simulink model "Modell_Slider_Regelung_Final"  (R2023a)
settings: Solver=FixedStepDiscrete  StartTime=0.0  StopTime=inf  FixedStep=0.1  RelTol=1e-3  EnableMultiTasking=on
model workspace (MAT data in the model file):
  value = 333.2859
undefined symbols (not defined in the file): HIL
libraries: quarc_library x4
settings Model: ExtModeTrigDuration=10000  Creator=Student  LastModifiedBy=Student
settings SolverCC: AlgebraicLoopSolver=TrustRegion  PositivePriorityOrder=on
settings DataIOCC: ReturnWorkspaceOutputs=off
settings DebuggingCC: UnconnectedInputMsg=warning  UnconnectedOutputMsg=warning  UnconnectedLineMsg=warning  ArithmeticOperatorsInVariantConditions=warning
settings ModelReferenceCC: EnableRefExpFcnMdlSchedulingChecks=on
settings SFSimCC: SimUseLocalCustomCode=off  CustomCodeUndefinedFunction=UseInterfaceOnly
settings RTWCC: Description=QUARC Win64 Target Using Toolchain  SystemTargetFile=quarc_win64.tlc  TemplateMakefile=quarc_default_tmf  RTWUseLocalCustomCode=off  Toolchain=QUARC win64 | nmake (64-bit Windows)  BuildConfiguration=Faster Runs
settings CodeAppCC: StateflowObjectComments=on
settings STFCustomTargetCC: SystemTargetFile=quarc_win64.tlc
settings GRTTargetCC: ParMdlRefBuildCompliant=off  CompOptLevelCompliant=off  CombineOutputUpdateFcns=off  MatFileLogging=off  CPPClassGenCompliant=off  GRTInterface=on  ExtMode=on  ExtModeMexFile=quarc_comm
settings ConfigComp: CovMetricSettings=dswe

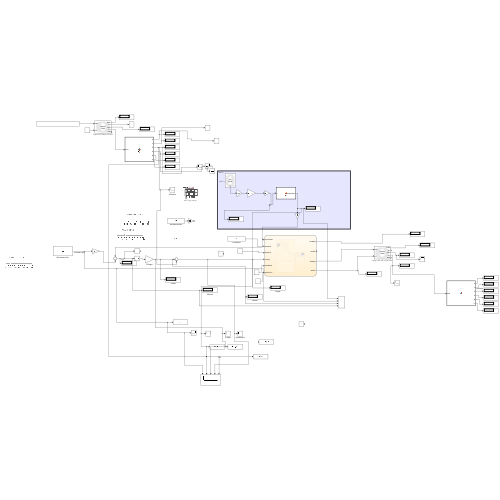
[thumbnail: Simulink's stored preview of the top-level diagram]
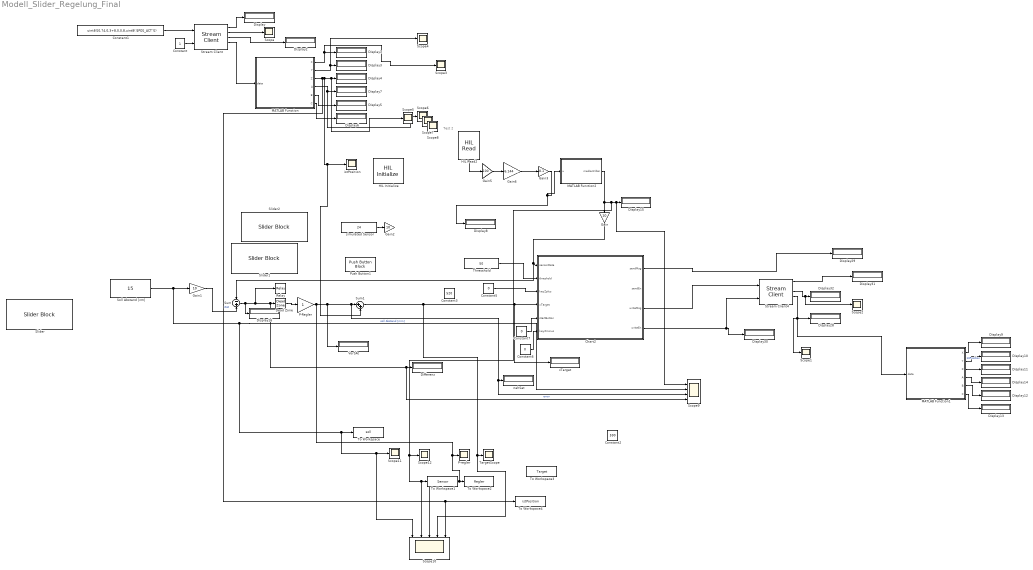
== system Modell_Slider_Regelung_Final ==
  note: Test 2
  Chart2 : Stateflow chart  TreatAsAtomicUnit=on
      settings: PortSchema="{\"entries\":[{\"content\":{\"sides\":[{\"content\":{\"connectorIds\":[\"In1\",\"In6\",\"In2\",\"In3\",\"In4\",\"In5\"]},\"type\":\"ConnectorPlacement.EquallySpacedRectSide\",\"uuid\":\"51d190bc-faf9-4413-9262-a39a5d664301\"},{\"content\":{\"connectorIds\":[\"Out1\",\"Out2\",\"Out3\",\"Out4\"],\"side\":\"RIGHT\"},\"type\":\"ConnectorPlacement.EquallySpacedRectSide\",\"uuid\":\"e4e93cb2-356d-4976-90dd-4fcabb178b84\"},{\"content\":{\"side\":\"TOP\"},\"type\":\"ConnectorPlacement.EquallySpacedRectSide\",\"uuid\":\"2a648fa8-8c40-468b-82f7-fe4bda6b12e2\"}]},\"type\":\"ConnectorPlacement.EquallySpacedConnector\",\"uuid\":\"c42a36e0-454c-4187-a45e-762c1b87647d\"}],\"packageUris\":[\"http://schema.mathworks.com/mf0/Connector/R2020b\"],\"version\":\"1.0\"}"
  Constant : Constant
  Constant1 : Constant  Value=uint8([0,74,0,3+8,0,0,8,uint8('$POS_ACT')])  OutDataTypeStr=uint8
  Constant2 : Constant  Value=590
  Constant3 : Constant  Value=520
  Constant5 : Constant  Value=0  OutDataTypeStr=boolean
  Constant6 : Constant  Value=0  OutDataTypeStr=boolean
  Constant7 : Constant  Value=0
  Dead Zone : DeadZone  LowerValue=-10  UpperValue=10
  Differenz : Display
  Display{,1..16,28..32} (22 alike) : Display
  Gain : Gain  Gain=10
  Gain1 : Gain  Gain=10
  Gain2 : Gain  Gain=10
  Gain3 : Gain  Gain=0.1
  Gain5 : Gain  Gain=100
  Gain6 : Gain  Gain=6.144
  HIL Initialize : quarc_library/Data Acquisition/Generic/Configuration/HIL Initialize  object_name=HIL-1  board_type=q2_usb  board_number=0  board_options=d0=digital;d1=digital;led=auto;update_rate=normal;decimation=1  exclusive=off  active=on  hardware_clocks=[0]  clock_modes=[]  initial_clock_frequencies=[]  set_clock_params_at_start=off  set_clock_params_at_switch_in=off  set_clock_frequencies_at_start=off  set_clock_frequencies_at_switch_in=off  analog_input_channels=[0:1]  analog_input_configurations=[]  analog_input_maximums=10  analog_input_minimums=-10  set_analog_input_params_at_start=on  set_analog_input_params_at_switch_in=off  analog_output_channels=[0:1]  analog_output_maximums=10  analog_output_minimums=-10  initial_analog_outputs=[0]  final_analog_outputs=[0]  watchdog_analog_outputs=0  set_analog_output_params_at_start=on  set_analog_output_params_at_switch_in=off  set_analog_outputs_at_start=on  set_analog_outputs_at_switch_in=off  set_analog_outputs_at_terminate=on  set_analog_outputs_at_switch_out=off  set_analog_outputs_on_watchdog=off  digital_input_channels=[]  digital_output_channels=[]  digital_output_configuration=[]  initial_digital_outputs=[1]  final_digital_outputs=[1]  watchdog_digital_outputs=[1]  set_digital_output_params_at_start=off  set_digital_output_params_at_switch_in=off  set_digital_outputs_at_start=on  set_digital_outputs_at_switch_in=off  set_digital_outputs_at_terminate=on  set_digital_outputs_at_switch_out=off  set_digital_outputs_on_watchdog=off  encoder_channels=[0:1]  quadrature=[4]  encoder_filter_frequency=[]  initial_encoder_counts=[0]  set_encoder_params_at_start=on  set_encoder_params_at_switch_in=off  set_encoder_counts_at_start=on  set_encoder_counts_at_switch_in=off  pwm_channels=[]  pwm_modes=[0]  pwm_frequency=1/0.020  pwm_configuration=[]  pwm_alignment=[]  pwm_polarity=[]  pwm_leading_deadband=[]  pwm_trailing_deadband=[]  initial_pwm_outputs=[0]  final_pwm_outputs=[0]  watchdog_pwm_outputs=[0]  set_pwm_params_at_start=on  set_pwm_params_at_switch_in=off  set_pwm_outputs_at_start=on  set_pwm_outputs_at_switch_in=off  set_pwm_outputs_at_terminate=on  set_pwm_outputs_at_switch_out=off  set_pwm_outputs_on_watchdog=off  other_output_channels=[]  initial_other_outputs=[]  final_other_outputs=[]  watchdog_other_outputs=[]  set_other_outputs_at_start=off  set_other_outputs_at_switch_in=off  set_other_outputs_at_terminate=off  set_other_outputs_at_switch_out=off  set_other_outputs_on_watchdog=off
  HIL Read2 : quarc_library/Data Acquisition/Generic/Immediate I//O/HIL Read  object_name=HIL-1  analog_channels=1  encoder_channels=[]  digital_channels=[]  other_channels=[]  sample_time=qc_get_step_size  active=on  vector_output=off  data_type_mode=Inherit via back propagation  encoder_data_type=double  digital_data_type=boolean
  MATLAB Function : MATLAB Function  TreatAsAtomicUnit=on
  MATLAB Function1 : MATLAB Function  TreatAsAtomicUnit=on
  MATLAB Function2 : MATLAB Function  TreatAsAtomicUnit=on
  P-Regler : Gain
  P-regler : Scope
  Push Button1 : PushButtonBlock  OffValue=0.000000
  Relay : Relay  OnSwitchValue=3  OffSwitchValue=1
  Scope{,1..8,11..12} (11 alike) : Scope
  Scope10 : Scope  NumInputPorts=5
  Scope9 : Scope  NumInputPorts=4
  Slider : SliderBlock  ScaleMax=80
  Slider1 : SliderBlock  ScaleMin=5  ScaleMax=150
  Slider2 : SliderBlock  ScaleMax=50
  Soll Abstand [cm] : Constant  Value=15
  Stream Client : quarc_library/Communications/Basic/Stream Client  uri_source=Specify via dialog (do not evaluate)  uri=tcpip://192.168.41.64:7000  send_buffer_size=1460  receive_buffer_size=1460  byte_order=little endian (Intel - LSB first)  optimization=Minimum latency  send_options=Send all data  receive_options=Receive all data  default_value=[uint8(0);uint8(0);uint8(0);uint8(0);uint8(0);uint8(0);uint8(0);uint8(0);uint8(0);uint8(0);uint8(0);uint8(0);uint8(0);uint8(0);uint8(0);uint8(0);uint8(0);uint8(0);uint8(0);uint8(0);uint8(0);uint8(0);uint8(0);uint8(0);uint8(0);uint8(0);uint8(0);uint8(0);uint8(0);uint8(0);uint8(0);uint8(0);uint8(0);uint8(0);uint8(0);uint8(0);uint8(0);uint8(0);uint8(0);uint8(0);uint8(0);uint8(0);uint8(0);uint8(0);uint8(0);uint8(0);uint8(0);uint8(0);uint8(0);uint8(0);uint8(0);uint8(0);uint8(0);uint8(0);uint8(0);uint8(0);uint8(0);uint8(0);uint8(0);uint8(0);uint8(0);uint8(0);uint8(0);uint8(0);uint8(0);uint8(0);uint8(0);uint8(0);uint8(0);uint8(0);uint8(0);uint8(0);uint8(0);uint8(0);uint8(0);uint8(0);uint8(0);uint8(0);uint8(0);uint8(0);uint8(0);uint8(0);uint8(0);uint8(0);uint8(0);uint8(0);uint8(0);uint8(0);uint8(0);uint8(0);uint8(0);uint8(0);uint8(0);uint8(0);uint8(0);uint8(0);uint8(0);uint8(0);uint8(0);uint8(0);uint8(0);uint8(0);uint8(0);uint8(0);uint8(0);uint8(0);uint8(0);uint8(0);uint8(0);uint8(0);uint8(0);uint8(0);uint8(0);uint8(0);uint8(0);uint8(0);uint8(0);uint8(0);uint8(0);uint8(0);uint8(0);uint8(0);uint8(0);uint8(0);uint8(0);uint8(0);uint8(0);uint8(0);uint8(0);uint8(0);uint8(0);uint8(0);uint8(0);uint8(0);uint8(0);uint8(0);uint8(0);uint8(0);uint8(0);uint8(0);uint8(0);uint8(0);uint8(0);uint8(0);uint8(0);uint8(0);uint8(0);uint8(0);uint8(0);uint8(0);uint8(0);uint8(0);uint8(0);uint8(0);uint8(0);uint8(0);uint8(0);uint8(0);uint8(0);uint8(0);uint8(0);uint8(0);uint8(0);uint8(0);uint8(0);uint8(0);uint8(0);uint8(0);uint8(0);uint8(0);uint8(0);uint8(0);uint8(0);uint8(0);uint8(0);uint8(0);uint8(0);uint8(0);uint8(0);uint8(0);uint8(0);uint8(0);uint8(0);uint8(0);uint8(0);uint8(0);uint8(0);uint8(0);uint8(0);uint8(0);uint8(0);uint8(0);uint8(0);uint8(0);uint8(0);uint8(0);uint8(0);uint8(0);uint8(0);uint8(0);uint8(0);uint8(0);uint8(0);uint8(0);uint8(0);uint8(0);uint8(0);uint8(0);uint8(0);uint8(0);uint8(0);uint8(0);uint8(0);uint8(0);uint8(0);uint8(0);uint8(0);uint8(0);uint8(0);uint8(0);uint8(0);uint8(0);uint8(0);uint8(0);uint8(0);uint8(0);uint8(0);uint8(0);uint8(0);uint8(0);uint8(0);uint8(0);uint8(0);uint8(0);uint8(0);uint8(0);uint8(0);uint8(0);uint8(0);uint8(0);uint8(0);uint8(0);uint8(0);uint8(0);uint8(0);uint8(0);uint8(0);uint8(0);uint8(0);uint8(0);uint8(0);uint8(0);uint8(0);uint8(0);uint8(0);uint8(0)]  sample_time=qc_get_step_size  active=off  implementation=Use blocking I/O in a separate thread  send_fifo_size=1000  receive_fifo_size=1000  send_priority=0  receive_priority=0  send_dimensions=off  receive_dimensions=off  max_dimensions=-1  data_type=uint8  type_expr=BusObject
      settings: AttributesFormatString="\"tcpip://192.168.41.64:7000\""
  Stream Client4 : quarc_library/Communications/Basic/Stream Client  uri_source=Specify via dialog (do not evaluate)  uri=tcpip://192.168.41.64:7000  send_buffer_size=1460  receive_buffer_size=1460  byte_order=little endian (Intel - LSB first)  optimization=Minimum latency  send_options=Send all data  receive_options=Receive all data  default_value=zeros(256,1,'uint8')  sample_time=qc_get_step_size  active=off  implementation=Use blocking I/O in a separate thread  send_fifo_size=1000  receive_fifo_size=1000  send_priority=0  receive_priority=0  send_dimensions=off  receive_dimensions=off  max_dimensions=-1  data_type=uint8  type_expr=BusObject
      settings: AttributesFormatString="\"tcpip://192.168.41.64:7000\""
  Sum : Sum  Inputs=-+
  Sum1 : Sum  Inputs=|++
  TargetScope : Scope
  Thresshold : Constant  Value=50
  To Workspace : ToWorkspace  VariableName=soll  SaveFormat=Structure With Time  SampleTime=-1
  To Workspace1 : ToWorkspace  VariableName=Sensor  SaveFormat=Structure With Time  SampleTime=-1
  To Workspace2 : ToWorkspace  VariableName=Regler  SaveFormat=Structure With Time  SampleTime=-1
  To Workspace3 : ToWorkspace  VariableName=Target  SaveFormat=Structure With Time  SampleTime=-1
  To Workspace4 : ToWorkspace  VariableName=istPosition  SaveFormat=Structure With Time  SampleTime=-1
  VorSAt : Display
  istPosition : Scope
  nahSat : Display
  simulated Sensor : Constant  Value=24
  xTarget : Display
  wires:
  Stream Client/1 -> Display/1
  Stream Client/2 -> Scope/1
  Constant1/1 -> Stream Client/1
  Stream Client/4 -> MATLAB Function/1(data)
  Stream Client/3 -> Display2/1
  MATLAB Function/1(X) -> Scope3/1, Display1/1
  MATLAB Function/4(A) -> Scope6/1, Display7/1
  MATLAB Function/5(B) -> Display5/1
  MATLAB Function/6(C) -> Display6/1
  Constant/1 -> Stream Client/2
  Stream Client4/3 -> Scope2/1, Display32/1
  Constant6/1 -> Chart2/5(keyZminus)
  Chart2/1(sendMsg) -> Display29/1
  Stream Client4/1 -> Display31/1
  Constant5/1 -> Chart2/2(keyZplus)
  Constant7/1 -> Chart2/4(startButton)
  Chart2/4(writeEn) -> Stream Client4/2, Display30/1
  Chart2/3(writeMsg) -> Stream Client4/1
  Gain5/1 -> Gain6/1
  HIL Read2/1 -> Gain5/1
  Gain6/1 -> Gain3/1
  Thresshold/1 -> Chart2/6(threshold)
  P-Regler/1 -> Scope10/3, To Workspace2/1, P-regler/1, Sum1/1, Scope9/3, nahSat/1, VorSAt/1
  MATLAB Function1/5(B) -> Display12/1
  MATLAB Function1/1(X) -> Display9/1
  Stream Client4/4 -> MATLAB Function1/1(data), Display28/1, Scope1/1
  MATLAB Function1/2(Y) -> Display10/1  "IstPosition"
  MATLAB Function1/3(Z) -> Display11/1
  MATLAB Function1/6(C) -> Display13/1
  MATLAB Function1/4(A) -> Display14/1
  Soll Abstand [cm]/1 -> Scope9/2, To Workspace/1, Scope10/1, Scope11/1, Gain1/1  "soll Abstand [mm]"
  Gain1/1 -> Sum/2
  simulated Sensor/1 -> Gain2/1
  MATLAB Function/2(Y) -> Scope4/1, Display3/1
  MATLAB Function2/1(medianFilter) -> Gain/1, To Workspace1/1, Scope10/2, Scope12/1, Scope9/1, Display15/1
  Gain3/1 -> Display8/1, MATLAB Function2/1(u)
  Dead Zone/1 -> P-Regler/1
  Gain/1 -> Sum/1, Chart2/1(sensorData)
  Sum1/1 -> Chart2/3(xTarget), xTarget/1, Scope10/4, TargetScope/1
  MATLAB Function/3(Z) -> Display4/1, Scope5/1, Sum1/2, istPosition/1, To Workspace4/1, Scope10/5  "Zist"
  Sum/1 -> Display16/1, Relay/1, Differenz/1, Scope9/4, Dead Zone/1  "error"

== matlab function Modell_Slider_Regelung_Final/MATLAB Function1 ==
  data: data input; X output; Y output; Z output; A output; B output; C output
function [X,Y,Z,A,B,C] = fcn(data)

% Standardwerte
X = NaN;
Y = NaN;
Z = NaN;
A = NaN;
B = NaN;
C = NaN;

% Empfangsdaten in einen Vektor umwandeln
data = data(:);

% Positionen suchen
ix = find(data == 88, 1, 'first');   % X
iy = find(data == 89, 1, 'first');   % Y
iz = find(data == 90, 1, 'first');   % Z
ia = find(data == 65, 1, 'first');   % A
ib = find(data == 66, 1, 'first');   % B
ic = find(data == 67, 1, 'first');   % C

% Zahlen auslesen
if ~isempty(ix)
    X = parseNumber(data, ix + 1);
end

if ~isempty(iy)
    Y = parseNumber(data, iy + 1);
end

if ~isempty(iz)
    Z = parseNumber(data, iz + 1);
end

if ~isempty(ia)
    A = parseNumber(data, ia + 1);
end

if ~isempty(ib)
    B = parseNumber(data, ib + 1);
end

if ~isempty(ic)
    C = parseNumber(data, ic + 1);
end

end


function value = parseNumber(data, startIndex)

value = 0;

n = numel(data);
idx = startIndex;

% Sicherstellen, dass idx ein Skalar ist
idx = idx(1);

% Leerzeichen überspringen
while idx <= n
    if data(idx) ~= 32
        break;
    end
    idx = idx + 1;
end

% Vorzeichen
sgn = 1;

if idx <= n
    if data(idx) == 45       % '-'
        sgn = -1;
        idx = idx + 1;
    elseif data(idx) == 43   % '+'
        idx = idx + 1;
    end
end

% Ganzzahlteil
while idx <= n
    if data(idx) < 48 || data(idx) > 57
        break;
    end

    value = value * 10 + double(data(idx) - 48);
    idx = idx + 1;
end

% Nachkommastellen
if idx <= n && data(idx) == 46       % '.'
    idx = idx + 1;

    factor = 0.1;

    while idx <= n
        if data(idx) < 48 || data(idx) > 57
            break;
        end

        value = value + double(data(idx) - 48) * factor;
        factor = factor * 0.1;
        idx = idx + 1;
    end
end

value = sgn * value;

end

== matlab function Modell_Slider_Regelung_Final/MATLAB Function ==
  data: data input; X output; Y output; Z output; A output; B output; C output
function [X,Y,Z,A,B,C] = fcn(data)

% Standardwerte
X = NaN;
Y = NaN;
Z = NaN;
A = NaN;
B = NaN;
C = NaN;

% Empfangsdaten in einen Vektor umwandeln
data = data(:);

% Positionen suchen
ix = find(data == 88, 1, 'first');   % X
iy = find(data == 89, 1, 'first');   % Y
iz = find(data == 90, 1, 'first');   % Z
ia = find(data == 65, 1, 'first');   % A
ib = find(data == 66, 1, 'first');   % B
ic = find(data == 67, 1, 'first');   % C

% Zahlen auslesen
if ~isempty(ix)
    X = parseNumber(data, ix + 1);
end

if ~isempty(iy)
    Y = parseNumber(data, iy + 1);
end

if ~isempty(iz)
    Z = parseNumber(data, iz + 1);
end

if ~isempty(ia)
    A = parseNumber(data, ia + 1);
end

if ~isempty(ib)
    B = parseNumber(data, ib + 1);
end

if ~isempty(ic)
    C = parseNumber(data, ic + 1);
end

end


function value = parseNumber(data, startIndex)

value = 0;

n = numel(data);
idx = startIndex;

% Sicherstellen, dass idx ein Skalar ist
idx = idx(1);

% Leerzeichen überspringen
while idx <= n
    if data(idx) ~= 32
        break;
    end
    idx = idx + 1;
end

% Vorzeichen
sgn = 1;

if idx <= n
    if data(idx) == 45       % '-'
        sgn = -1;
        idx = idx + 1;
    elseif data(idx) == 43   % '+'
        idx = idx + 1;
    end
end

% Ganzzahlteil
while idx <= n
    if data(idx) < 48 || data(idx) > 57
        break;
    end

    value = value * 10 + double(data(idx) - 48);
    idx = idx + 1;
end

% Nachkommastellen
if idx <= n && data(idx) == 46       % '.'
    idx = idx + 1;

    factor = 0.1;

    while idx <= n
        if data(idx) < 48 || data(idx) > 57
            break;
        end

        value = value + double(data(idx) - 48) * factor;
        factor = factor * 0.1;
        idx = idx + 1;
    end
end

value = sgn * value;

end

== matlab function Modell_Slider_Regelung_Final/MATLAB Function2 ==
  data: u input; medianFilter output
function medianFilter = fcn(u)
    persistent iWrite  buffer counter ;
    
    window_length = 10
    u = fix(u)

    if isempty(buffer)
        buffer = zeros(window_length,1)
        iWrite = 1
        counter = 0
    end
    
    buffer(iWrite) = u
    iWrite = iWrite +1
    counter = counter + 1
    
    
    if iWrite > window_length
        iWrite = 1
    end


    if counter > window_length
        counter = window_length;
    end
    
    
    
    
     medianFilter = fix(median(buffer(1:counter)));

end

== stateflow chart Modell_Slider_Regelung_Final/Chart2 ==
  state Superstate
    state IDLE
      entry:
      writeEn = false;
    state INIT_END
      entry:
      writeMsg = buildEndTrueMsg();
      writeEn = true;
    state WAIT_END
      entry:
      writeEn= false;
    state SET_MODE
      entry:
      writeMsg = buildMode3Msg();
      writeEn = true;
    state WAIT_MODE
      entry:
      writeEn = false;
    state HOLD
      entry:
      writeEn = false;
    state STOP_MOVE
      entry:
      writeMsg = buildEndTrueMsg();
      writeEn = true;
    (default) -> IDLE
    HOLD -> IDLE : [~startButton]
    IDLE -> INIT_END : [startButton]
    INIT_END -> WAIT_END : after(1,tick)
    WAIT_END -> SET_MODE : after(30,tick)
    SET_MODE -> WAIT_MODE : after(1,tick)
    WAIT_MODE -> (junction 188) : after(10,tick)
    (junction 188) -> STOP_MOVE [order 1] : [threshold > sensorData
        | ]
    STOP_MOVE -> HOLD : after(1,tick)
  state Moving
    state START_MOVE
      entry:
      writeMsg = buildEndFalseMsg();
      writeEn = true;
    state MOVE_STEP
      entry:
      writeMsg = buildTargetMsg(xTarget);
      writeEn  = true;
    state WRITE_P1 [commented out]
      entry:
      writeMsg = buildTargetMsg(zTarget);
      writeEn = true;
    state WAIT_P1 [commented out]
      entry:
      writeEn = false;
    (default) -> START_MOVE
    START_MOVE -> MOVE_STEP : after(1,tick)
    (junction 191) -> MOVE_STEP [order 2] : after(30, tick)
    MOVE_STEP -> (junction 191)
    (default) -> WRITE_P1 [commented out]
  (default) -> Superstate
  (junction 188) -> START_MOVE [order 2]
  (junction 191) -> STOP_MOVE [order 1] : [threshold > sensorData
      | ]
  Moving -> STOP_MOVE : [threshold > sensorData
      | ]
  data: msg function_output; msg function_output; msg function_output; xTarget function_input; msg function_output; sensorData input; sendMsg output uint8 size=[1 21]; sendEn output boolean size=[1]; msgKeyZminus constant uint8 size=[1 21] =uint8([0,5,0,14,1,0,7,uint8('KEYFLAG'),0,2,uint8('05'),0,0,0]); msgKeyZplus constant uint8 size=[1 21] =uint8([0,6,0,14,1,0,7,uint8('KEYFLAG'),0,2,uint8('06'),0,0,0]); msgKey0 constant uint8 size=[1 21] =uint8([0,21,0,13,1,0,7,uint8('KEYFLAG'),0,1,uint8('0'),0,0,0,0]); msgActOn constant uint8 size=[1 21] =uint8([0,60,0,16,1,0,7,uint8('ACTFLAG'),0,4,uint8('TRUE'),0]); msgActOff constant uint8 size=[1 21] =uint8([0,60,0,17,1,0,7,uint8('ACTFLAG'),0,5,uint8('FALSE')]); activeKey local uint8 =0; prevZplus local boolean size=[1]; prevZminus local boolean size=[1]; keyZplus input boolean size=[1]; xTarget input double size=1; startButton input; keyZminus input boolean size=[1]; fallActive local boolean size=[1]; riseZminus local boolean size=[1]; riseZplus local boolean size=[1]; writeMsg output uint8 size=[1 256]; writeEn output; data local; data1 local; threshold input; data3 local; dx local double =2
  data dx settings: description=weg schritte um Fahrt zu stoppen
  function msg= buildEndTrueMsg:
    | function msg= buildEndTrueMsg()
    | 
    | msg = uint8([0,20, ...
    |     0,16, 1,0,7, uint8('ENDPROG'), 0,4 , uint8('TRUE')]);
    | 
    | end
  function msg = buildMode3Msg:
    | function msg = buildMode3Msg()
    | 
    | progmsg = uint8([ ...
    |     0,30, ...
    |     0,13, ...
    |     1, ...
    |     0,7, ...
    |     uint8('PROGVAR'), ...
    |     0,1, ...
    |     uint8('3')]);
    | 
    | actmsg = uint8([ ...
    |     0,60, ...
    |     0,16, ...
    |     1, ...
    |     0,7, ...
    |     uint8('ACTFLAG'), ...
    |     0,4, ...
    |     uint8('TRUE')]);
    | 
    | endmsg = uint8([ ...
    |     0,20, ...
    |     0,16, ...
    |     1, ...
    |     0,7, ...
    |     uint8('ENDPROG'), ...
    |     0,4, ...
    |     uint8('TRUE')]);
    | 
    | msg = [progmsg, actmsg, endmsg];
    | 
    | end
  function msg = buildTargetMsg(xTarget):
    | function msg = buildTargetMsg(xTarget)
    | 
    | x = 427; %427
    | y = 54.02;%
    | z = xTarget;%574
    | a = 90;%90
    | b = 89;%89
    | c = 90;%90
    | s = int32(2);
    | t = int32(42);
    | 
    | tempChar = sprintf( ...
    |     '{POS: X %.1f,Y %.1f,Z %.1f,A %.1f,B %.1f,C %.1f,S %d,T %d}', ...
    |     x,y,z,a,b,c,s,t);
    | 
    | temp = uint8(tempChar);
    | 
    | msg = uint8([ ...
    |     0,13, ...
    |     0,3+8+length(temp)+2, ...
    |     1, ...
    |     0,8, ...
    |     uint8('MAT_POS1'), ...
    |     0,length(temp), ...
    |     temp]);
    | 
    | end
  function msg = buildEndFalseMsg:
    | function msg = buildEndFalseMsg()
    | 
    | msg = uint8([0,20 ,0 ,17,1,0,7,uint8('ENDPROG'),0,5,uint8('FALSE')]);
    | 
    | end
